simulink model "FTVsWBD_SingleSupportLefttLeg"  (R2014a)
settings: Solver=FixedStepDiscrete  StartTime=0.0  StopTime=5  FixedStep=Ts  RelTol=1e-3
undefined symbols (not defined in the file): localName, robotName, Ts
libraries: WBCLibrary x3
settings Model: Creator=jorhabib  LastModifiedBy=jorhabib

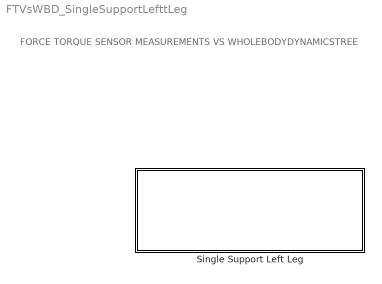
== system FTVsWBD_SingleSupportLefttLeg ==
  note: FORCE TORQUE SENSOR MEASUREMENTS
      |                                   VS
      |              WHOLEBODYDYNAMICSTREE
  Single Support Left Leg : Subsystem  mask{robotName=robotName, localName=localName, Ts=Ts}
      mask prompts: robotName "Robot Name"; localName "Local Name"; Ts "Simulation Period"

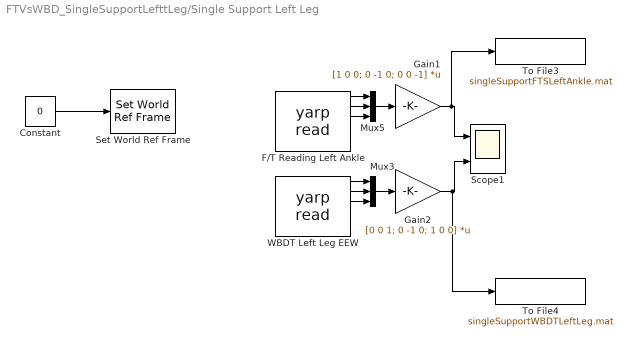
== system FTVsWBD_SingleSupportLefttLeg/Single Support Left Leg ==
  Constant : Constant  Value=0  OutDataTypeStr=int8
  F/T Reading Left Ankle : WBCLibrary/Utilities/yarp read  from=['/icub' '/left_foot/analog:o']  to='...'  num=6
  Gain1 : Gain  Gain=[1 0 0; 0 -1 0; 0 0 -1]  Multiplication=Matrix(K*u)
  Gain2 : Gain  Gain=[0 0 1; 0 -1 0; 1 0 0]  Multiplication=Matrix(K*u)
  Mux3 : Mux  Inputs=3
  Mux5 : Mux  Inputs=3
  Scope1 : Scope  NumInputPorts=2
      settings: YMin=40~-30  YMax=130~140
  Set World Ref Frame : WBCLibrary/wholeBodyModel/Set World Ref Frame  robotName=robotName  localName=localName
  To File3 : ToFile  Filename=singleSupportFTSLeftAnkle.mat  MatrixName=singleSupportFTSLeftAnkle  SaveFormat=Timeseries  SampleTime=Ts
  To File4 : ToFile  Filename=singleSupportWBDTLeftLeg.mat  MatrixName=singleSupportWBDTLeftLeg  SaveFormat=Timeseries
  WBDT Left Leg EEW : WBCLibrary/Utilities/yarp read  from=['/wholeBodyDynamicsTree' '/left_leg/endEffectorWrench:o']  to='...'  num=6
  wires:
  Mux3/1 -> Gain2/1
  Mux5/1 -> Gain1/1
  WBDT Left Leg EEW/3 -> Mux3/3
  WBDT Left Leg EEW/2 -> Mux3/2
  WBDT Left Leg EEW/1 -> Mux3/1
  F/T Reading Left Ankle/3 -> Mux5/3
  F/T Reading Left Ankle/2 -> Mux5/2
  F/T Reading Left Ankle/1 -> Mux5/1
  Gain2/1 -> Scope1/2, To File4/1
  Gain1/1 -> Scope1/1, To File3/1
  Constant/1 -> Set World Ref Frame/1
